simulink model "t2_sim_auto"  (Simulink 7.3)
settings: Solver=ode45  StartTime=0.0  StopTime=4  RelTol=1e-3
values from neighbouring files (symbols this model uses):
  B = 5    [t1.m]
  K = 50    [t1.m]
  kd = 5    [t1.m]
  kp = 2547    [t1.m]
  kv = 0    [t1.m]
  M = 1    [t1.m]
  Ts = .02    (= 0.02)    [t1.m]
libraries: sdolib x1
settings Model: Creator=arash  LastModifiedBy=arash

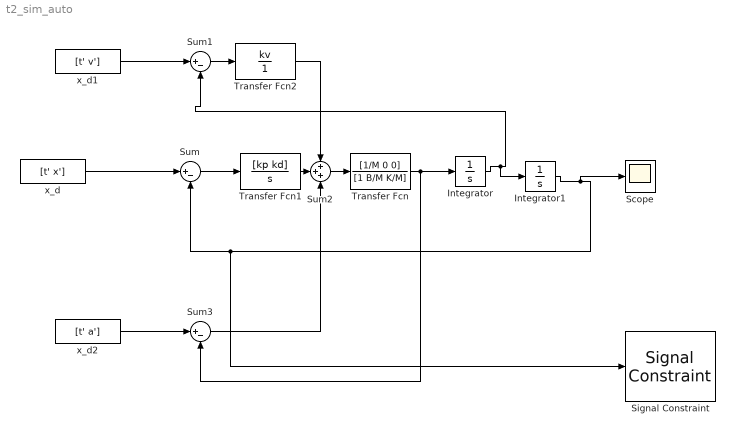
== system t2_sim_auto ==
  Integrator : Integrator
  Integrator1 : Integrator
  Scope : Scope
      settings: TimeRange=15
  Signal Constraint : sdolib/Signal Constraint  SystemSampleTime=-1  DialogPosition=[1.13828125 0.18875 0.45 0.31]  SaveIn=workspace  LogID=SRO_DataLog_1
  Sum : Sum  Inputs=|+-  OutDataType=fixdt(1, 16)  OutScaling=2^0
  Sum1 : Sum  Inputs=|+-  OutDataType=fixdt(1, 16)  OutScaling=2^0
  Sum2 : Sum  Inputs=+++  OutDataType=fixdt(1, 16)  OutScaling=2^0
  Sum3 : Sum  Inputs=|+-  OutDataType=fixdt(1, 16)  OutScaling=2^0
  Transfer Fcn : TransferFcn  Numerator=[1/M 0 0]  Denominator=[1 B/M K/M]
  Transfer Fcn1 : TransferFcn  Numerator=[kp kd]  Denominator=[1 0]
  Transfer Fcn2 : TransferFcn  Numerator=kv  Denominator=1
  x_d : FromWorkspace  VariableName=[t' x']  SampleTime=Ts
  x_d1 : FromWorkspace  VariableName=[t' v']  SampleTime=Ts
  x_d2 : FromWorkspace  VariableName=[t' a']  SampleTime=Ts
  wires:
  Sum/1 -> Transfer Fcn1/1
  x_d/1 -> Sum/1
  Transfer Fcn/1 -> Integrator/1, Sum3/2
  Sum2/1 -> Transfer Fcn/1
  Transfer Fcn1/1 -> Sum2/2
  x_d1/1 -> Sum1/1
  Integrator1/1 -> Scope/1, Sum/2, Signal Constraint/1
  Integrator/1 -> Sum1/2, Integrator1/1
  x_d2/1 -> Sum3/1
  Sum1/1 -> Transfer Fcn2/1
  Transfer Fcn2/1 -> Sum2/1
  Sum3/1 -> Sum2/3
